simulink model "roll"  (R2024b)
settings: Solver=VariableStepAuto  StartTime=0.0  StopTime=0.2  RelTol=1e-3
model workspace (MAT data in the model file):
  I = 5.94e-05
  b = 1
settings Model: Creator=Zohaib  LastModifiedBy=Zohaib

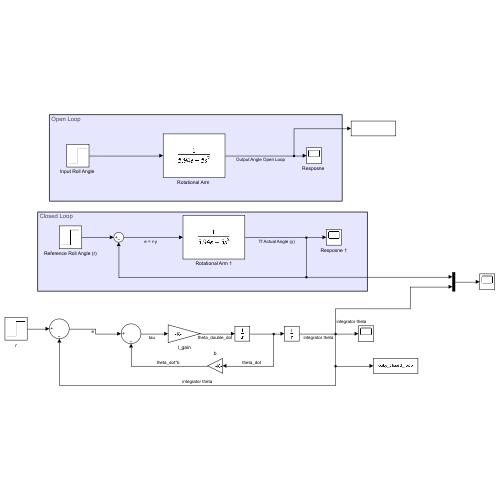
[thumbnail: Simulink's stored preview of the top-level diagram]
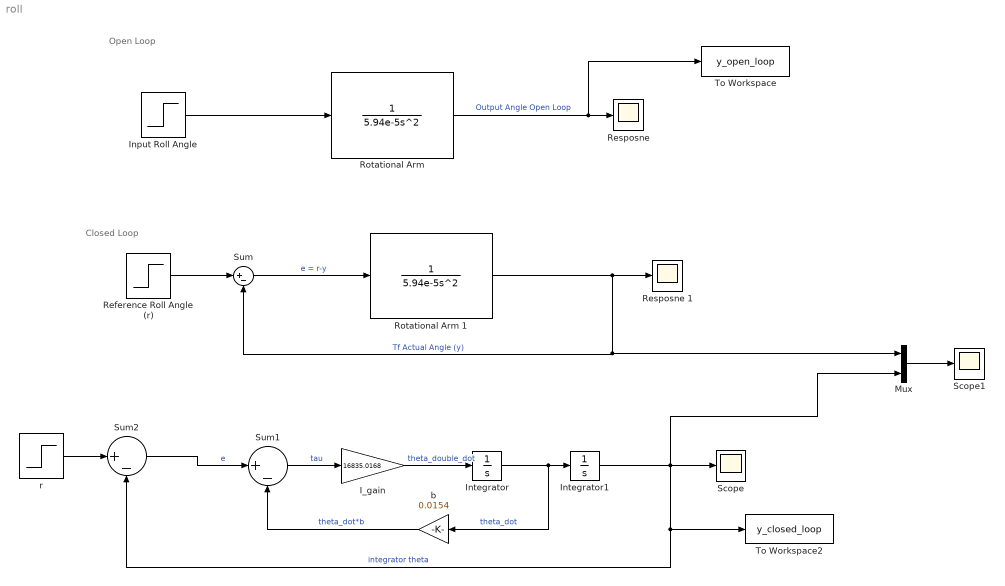
== system roll ==
  note: Closed Loop
  note: Open Loop
  I_gain : Gain  Gain=16835.0168
  "Input Roll Angle " : Step  SampleTime=0
  Integrator : Integrator
  Integrator1 : Integrator
  Mux : Mux  Inputs=2
  Reference Roll Angle (r) : Step  Time=0  SampleTime=0
  "Resposne " : Scope
  Resposne 1 : Scope
  "Rotational Arm " : TransferFcn  Denominator=[5.94e-5 0 0]
  Rotational Arm 1 : TransferFcn  Denominator=[5.94e-5 0 0]
  Scope : Scope
  Scope1 : Scope
  Sum : Sum  Inputs=|+-
  Sum1 : Sum  Inputs=|+-
  Sum2 : Sum  Inputs=|+-
  To Workspace : ToWorkspace  VariableName=y_open_loop  SaveFormat=Timeseries  SampleTime=-1
  To Workspace2 : ToWorkspace  VariableName=y_closed_loop  SaveFormat=Timeseries  SampleTime=-1
  b : Gain  Gain=0.0154
  r : Step  Time=0  After=5*(pi/180)  SampleTime=0
  wires:
  "Input Roll Angle "/1 -> "Rotational Arm "/1
  "Rotational Arm "/1 -> To Workspace/1, "Resposne "/1  "Output Angle Open Loop"
  Rotational Arm 1/1 -> Sum/2, Mux/1, Resposne 1/1  "Tf Actual Angle (y)"
  Reference Roll Angle (r)/1 -> Sum/1
  Sum/1 -> Rotational Arm 1/1  "e = r-y"
  Sum1/1 -> I_gain/1  "tau"
  I_gain/1 -> Integrator/1  "theta_double_dot"
  Integrator/1 -> b/1, Integrator1/1  "theta_dot"
  Integrator1/1 -> Scope/1, Mux/2, To Workspace2/1, Sum2/2  "integrator theta"
  b/1 -> Sum1/2  "theta_dot*b"
  r/1 -> Sum2/1
  Sum2/1 -> Sum1/1  "e"
  Mux/1 -> Scope1/1
